simulink subsystem "mission_supervisor_sys"  (R2020a)
settings: Solver=VariableStepAuto  StartTime=0.0  StopTime=10.0  RelTol=1e-3
values from neighbouring files (symbols this model uses):
  bool_inspection = 1    [initCheckpoints.m]
  checkpoints = [M100; M201; M202]    [initCheckpoints.m]
  counter_max = max(size(M201,1),size(M202,1))    [initCheckpoints.m]
libraries: simulink x1
settings Model: Creator=andrea  LastModifiedBy=pietro

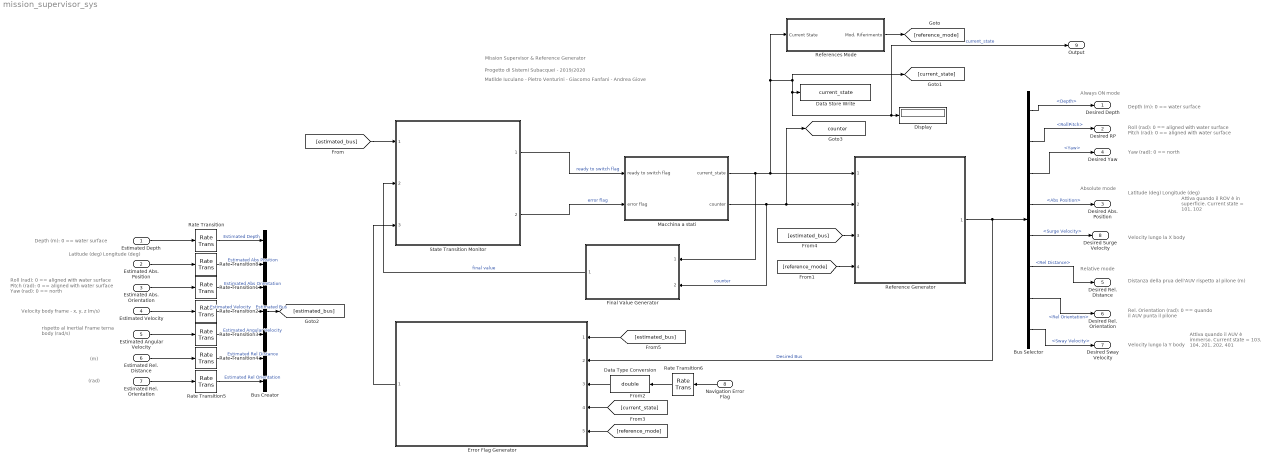
== system mission_supervisor_sys ==
  note: Velocity lungo la X body
  note: Depth (m): 0 == water surface
  note: Attiva quando il ROV è in superficie.
      | Current state = 101, 102
  note: (rad)
  note: (m)
  note: Always ON mode
  note: Relative mode
  note: Roll (rad): 0 == aligned with water surface
      | Pitch (rad): 0 == aligned with water surface
  note: Absolute mode
  note: Depth (m): 0 == water surface
  note: Latitude (deg)
      | Longitude (deg)
  note: Latitude (deg)
      | Longitude (deg)
  note: Roll (rad): 0 == aligned with water surface
      | Pitch (rad): 0 == aligned with water surface
      | Yaw (rad): 0 == north
  note: Velocity body frame - x, y, z (m/s)
  note: rispetto al Inertial Frame
      | terna body
      | (rad/s)
  note: Distanza della prua dell'AUV rispetto al pilone (m)
  note: Yaw (rad): 0 == north
  note: Rel. Orientation (rad):
      | 0 == quando il AUV punta il pilone
  note: Velocity lungo la Y body
  note: Attiva quando il AUV è immerso.
      | Current state = 103, 104, 201, 202, 401
  note: Mission Supervisor & Reference Generator
  note: Progetto di Sistemi Subacquei - 2019/2020
  note: Matilde Iuculano - Pietro Venturini - Giacomo Fanfani - Andrea Giove
  Estimated Depth : Inport
  Estimated Abs. Position : Inport  Port=2
  Estimated Abs. Orientation : Inport  Port=3
  Estimated Velocity : Inport  Port=4
  Estimated Angular Velocity : Inport  Port=5
  Estimated Rel. Distance : Inport  Port=6
  Estimated Rel. Orientation : Inport  Port=7
  Navigation Error Flag : Inport  Port=8
  Bus Creator : BusCreator  Inputs=7
  Bus Selector : BusSelector  OutputSignals=Depth,RollPitch,Yaw,Abs Position,Surge Velocity,Rel Distance,Rel Orientation,Sway Velocity
  Data Store Write : DataStoreWrite  DataStoreName=current_state
  Data Type Conversion : DataTypeConversion  OutDataTypeStr=double
  Display : Display
  Error Flag Generator : Subsystem  ReferencedSubsystem=error_flag_generator
  "Final Value Generator " : Subsystem  ReferencedSubsystem=final_value_generator  checkpoints=checkpoints  counter_max=length_201
  Macchina a stati : Subsystem
  Rate Transition{,1..6,8} (8 alike) : RateTransition  Deterministic=off  OutPortSampleTime=misu_Ts
  Reference Generator : Subsystem  ReferencedSubsystem=reference_generator  x_params=checkpoints(:,[1,5,9])  y_params=checkpoints(:,[2,6,10])  depth_params=checkpoints(:,[3,7,11])  abs_yaw_params=checkpoints(:,[4,8,12])  distance=distance  desired_lat_vel=speed  lat_vel_error_gain=1  counter_max=length_201
  References Mode : Subsystem
  State Transition Monitor : Subsystem  ReferencedSubsystem=state_transition_monitor
  Desired Depth : Outport
  Desired RP : Outport  Port=2
  Desired Abs. Position : Outport  Port=3
  Desired Yaw : Outport  Port=4
  Desired Rel. Distance : Outport  Port=5
  Desired Rel. Orientation : Outport  Port=6
  Desired Sway Velocity : Outport  Port=7
  Desired Surge Velocity : Outport  Port=8
  Output : Outport  Port=9
  tag scope: counter=global
  wires:
  Estimated Depth/1 -> Rate Transition/1
  Estimated Abs. Position/1 -> Rate Transition8/1
  Estimated Abs. Orientation/1 -> Rate Transition1/1
  Estimated Velocity/1 -> Rate Transition2/1
  Estimated Angular Velocity/1 -> Rate Transition3/1
  Estimated Rel. Distance/1 -> Rate Transition4/1
  Estimated Rel. Orientation/1 -> Rate Transition5/1
  References Mode/1(Mod. Riferimento) -> [reference_mode]
  Error Flag Generator/1 -> State Transition Monitor/3
  Bus Creator/1 -> [estimated_bus]  "Estimated Bus"
  Navigation Error Flag/1 -> Rate Transition6/1
  Reference Generator/1 -> Error Flag Generator/2, Bus Selector/1  "Desired Bus"
  Bus Selector/1 -> Desired Depth/1  "<Depth>"
  Bus Selector/2 -> Desired RP/1  "<RollPitch>"
  Bus Selector/4 -> Desired Abs. Position/1  "<Abs Position>"
  Bus Selector/3 -> Desired Yaw/1  "<Yaw>"
  Bus Selector/6 -> Desired Rel. Distance/1  "<Rel Distance>"
  Bus Selector/7 -> Desired Rel. Orientation/1  "<Rel Orientation>"
  Bus Selector/8 -> Desired Sway Velocity/1  "<Sway Velocity>"
  "Final Value Generator "/1 -> State Transition Monitor/2  "final value"
  Macchina a stati/2(counter) -> "Final Value Generator "/2, Reference Generator/2, [counter]  "counter"
  Macchina a stati/1(current_state) -> Reference Generator/1, [current_state], Data Store Write/1, Display/1, Output/1, References Mode/1(Current State), "Final Value Generator "/1  "current_state"
  [reference_mode] -> Reference Generator/4
  State Transition Monitor/2 -> Macchina a stati/2(error flag)  "error flag"
  State Transition Monitor/1 -> Macchina a stati/1(ready to switch flag)  "ready to switch flag"
  Bus Selector/5 -> Desired Surge Velocity/1  "<Surge Velocity>"
  [current_state] -> Error Flag Generator/4
  [reference_mode] -> Error Flag Generator/5
  [estimated_bus] -> State Transition Monitor/1
  [estimated_bus] -> Reference Generator/3
  [estimated_bus] -> Error Flag Generator/1
  Rate Transition/1 -> Bus Creator/1  "Estimated Depth"
  Rate Transition8/1 -> Bus Creator/2  "Estimated Abs Position"
  Rate Transition1/1 -> Bus Creator/3  "Estimated Abs Orientation"
  Rate Transition2/1 -> Bus Creator/4  "Estimated Velocity"
  Rate Transition3/1 -> Bus Creator/5  "Estimated Angular Velocity"
  Rate Transition4/1 -> Bus Creator/6  "Estimated Rel Distance"
  Rate Transition5/1 -> Bus Creator/7  "Estimated Rel Orientation"
  Rate Transition6/1 -> Data Type Conversion/1
  Data Type Conversion/1 -> Error Flag Generator/3

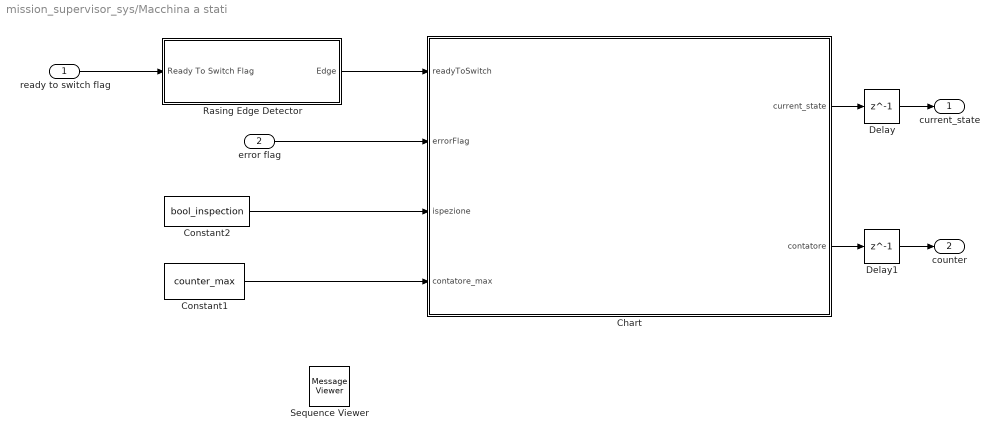
== system mission_supervisor_sys/Macchina a stati ==
  ready to switch flag : Inport
  error flag : Inport  Port=2
  Chart : Stateflow chart  TreatAsAtomicUnit=on
  Constant1 : Constant  Value=counter_max
  Constant2 : Constant  Value=bool_inspection
  Delay : Delay  DelayLength=1
  Delay1 : Delay  DelayLength=1
  Rasing Edge Detector : Subsystem
  Sequence Viewer : MessageViewer  History=1000  SavedRootId=#
  current_state : Outport
  counter : Outport  Port=2
  wires:
  Constant2/1 -> Chart/3(ispezione)
  Constant1/1 -> Chart/4(contatore_max)
  Rasing Edge Detector/1(Edge) -> Chart/1(readyToSwitch)
  ready to switch flag/1 -> Rasing Edge Detector/1(Ready To Switch Flag)
  error flag/1 -> Chart/2(errorFlag)
  Chart/1(current_state) -> Delay/1
  Chart/2(contatore) -> Delay1/1
  Delay1/1 -> counter/1
  Delay/1 -> current_state/1

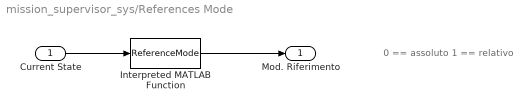
== system mission_supervisor_sys/References Mode ==
  note: 0 == assoluto
      | 1 == relativo
  Current State : Inport
  Interpreted MATLAB Function : MATLABFcn  MATLABFcn=ReferenceMode
  Mod. Riferimento : Outport
  wires:
  Interpreted MATLAB Function/1 -> Mod. Riferimento/1
  Current State/1 -> Interpreted MATLAB Function/1

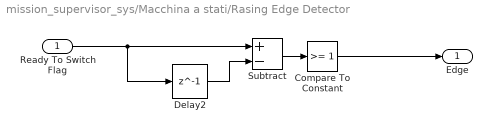
== system mission_supervisor_sys/Macchina a stati/Rasing Edge Detector ==
  Ready To Switch Flag : Inport
  Compare To Constant : simulink/Logic and Bit Operations/Compare To Constant  relop=>=  const=1  OutDataTypeStr=boolean
  Delay2 : Delay  DelayLength=1
  Subtract : Sum  Inputs=+-
  Edge : Outport
  wires:
  Ready To Switch Flag/1 -> Delay2/1, Subtract/1
  Compare To Constant/1 -> Edge/1
  Subtract/1 -> Compare To Constant/1
  Delay2/1 -> Subtract/2

== stateflow chart mission_supervisor_sys/Macchina a stati/Chart ==
  state START
    current_state=0;
    contatore=0;
  state ISPEZIONE
    state FASE_DI_PREISPEZIONE
      contatore = 0;
      state SCELTA_MISSIONE
    state ISPEZIONE_VERTICALE
      state ARCO_DI_CIRCONFERENZA
        current_state = 202
      state SALITA_DISCESA
        current_state= 201
      ISPEZIONE.ISPEZIONE_VERTICALE.SALITA_DISCESA -> ISPEZIONE.ISPEZIONE_VERTICALE.ARCO_DI_CIRCONFERENZA [order 1] : [readyToSwitch]
      ISPEZIONE.ISPEZIONE_VERTICALE.ARCO_DI_CIRCONFERENZA -> ISPEZIONE.ISPEZIONE_VERTICALE.SALITA_DISCESA : [readyToSwitch]{contatore = contatore + 1}
    state ISPEZIONE_ORIZZONTALE
      state ARCO_DI_CIRCONFERENZA
        current_state = 202
      state SALITA_DISCESA
        current_state= 201
      ISPEZIONE.ISPEZIONE_ORIZZONTALE.ARCO_DI_CIRCONFERENZA -> ISPEZIONE.ISPEZIONE_ORIZZONTALE.SALITA_DISCESA [order 1] : [readyToSwitch]
      ISPEZIONE.ISPEZIONE_ORIZZONTALE.SALITA_DISCESA -> ISPEZIONE.ISPEZIONE_ORIZZONTALE.ARCO_DI_CIRCONFERENZA : [readyToSwitch]{contatore = contatore + 1}
    SCELTA_MISSIONE -> ISPEZIONE.ISPEZIONE_ORIZZONTALE.ARCO_DI_CIRCONFERENZA [order 1] : [ispezione==0]
    SCELTA_MISSIONE -> ISPEZIONE.ISPEZIONE_VERTICALE.SALITA_DISCESA [order 2] : [ispezione]
  state INIZIALIZZAZIONE
    state TRAIETTORIA
      current_state = 102;
    state ROTAZIONE_SUL_POSTO
      current_state = 101;
    state IMMERSIONE
      current_state = 104;
    state ROTAZIONE_INTORNO_AL_PILONE
      current_state = 103;
    (default) -> ROTAZIONE_SUL_POSTO
    ROTAZIONE_SUL_POSTO -> TRAIETTORIA : [readyToSwitch]
    TRAIETTORIA -> ROTAZIONE_INTORNO_AL_PILONE : [[readyToSwitch]]
    ROTAZIONE_INTORNO_AL_PILONE -> IMMERSIONE : [readyToSwitch]
  state Change_Step
  state RITORNO_IN_SUPERFICIE
    state RISALITA_IN_SUPERFICIE
      current_state = 401;
  state ERRORE
    current_state = 500;
    contatore=0;
  state FINE_MISSIONE
    current_state=999;
  Change_Step -> RISALITA_IN_SUPERFICIE : [readyToSwitch]{contatore=0;}
  IMMERSIONE -> SCELTA_MISSIONE : [readyToSwitch]
  RISALITA_IN_SUPERFICIE -> FINE_MISSIONE : [readyToSwitch]
  ISPEZIONE.ISPEZIONE_ORIZZONTALE.ARCO_DI_CIRCONFERENZA -> Change_Step [order 2] : [contatore == contatore_max - 1]
  ISPEZIONE.ISPEZIONE_VERTICALE.SALITA_DISCESA -> Change_Step [order 2] : [contatore == contatore_max - 1]
  (default) -> START
  START -> INIZIALIZZAZIONE
  INIZIALIZZAZIONE -> ERRORE : [errorFlag]
  ISPEZIONE -> ERRORE : [errorFlag]
  FINE_MISSIONE -> ERRORE : [errorFlag]
  RITORNO_IN_SUPERFICIE -> ERRORE : [errorFlag]
  data: readyToSwitch input; current_state output; contatore output; errorFlag input; ispezione input; contatore_max input double
